simulink model "PTn_model_Z1"  (R2024a)
settings: Solver=ode45  StartTime=0.0  StopTime=20.0  FixedStep=1e-2  RelTol=1e-4  AbsTol=1e-4
values from neighbouring files (symbols this model uses):
  den = [1, 2*D, 1]    [ITAE_Plots_PT2_Schwingfaehig.m]    (also in ITAE_Plots_PTn.m = den_list{i})
  Kp = pid_params{i,j}(1)    [ITAE_Plots_PT2_Schwingfaehig.m]    (also in ITAE_Plots_PTn.m)
  lower_limit = limits(j,2)    [ITAE_Plots_PT2_Schwingfaehig.m]    (also in ITAE_Plots_PTn.m)
  num = [1]    [ITAE_Plots_PT2_Schwingfaehig.m]    (also in ITAE_Plots_PTn.m)
  Tn = pid_params{i,j}(2)    [ITAE_Plots_PT2_Schwingfaehig.m]    (also in ITAE_Plots_PTn.m)
  Tv = pid_params{i,j}(3)    [ITAE_Plots_PT2_Schwingfaehig.m]    (also in ITAE_Plots_PTn.m)
  upper_limit = limits(j,1)    [ITAE_Plots_PT2_Schwingfaehig.m]    (also in ITAE_Plots_PTn.m)
settings Model: Creator=bhir  LastModifiedBy=Flo
settings SolverCC: AlgebraicLoopSolver=TrustRegion
settings DataIOCC: ReturnWorkspaceOutputs=off
settings DebuggingCC: UnconnectedInputMsg=warning  UnconnectedOutputMsg=warning  UnconnectedLineMsg=warning  ArithmeticOperatorsInVariantConditions=warning
settings SFSimCC: SimUseLocalCustomCode=off  CustomCodeUndefinedFunction=UseInterfaceOnly
settings RTWCC: RTWUseLocalCustomCode=off  GPUComputeCapability=3.5  DLArmComputeVersion=19.05
settings CodeAppCC: StateflowObjectComments=on

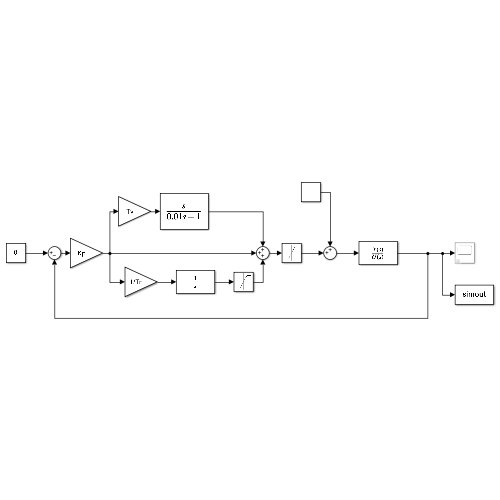
[thumbnail: Simulink's stored preview of the top-level diagram]
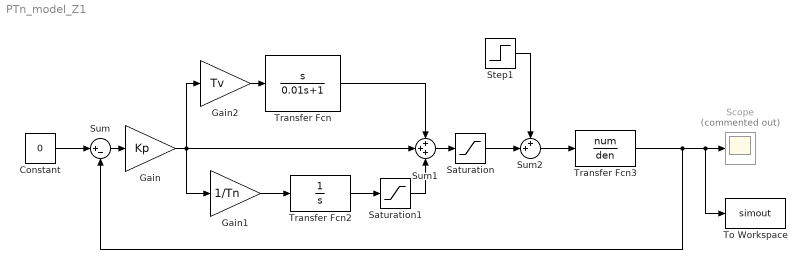
== system PTn_model_Z1 ==
  Constant : Constant  Value=0
  Gain : Gain  Gain=Kp
  Gain1 : Gain  Gain=1/Tn
  Gain2 : Gain  Gain=Tv
  Saturation : Saturate  UpperLimit=upper_limit  LowerLimit=lower_limit
  Saturation1 : Saturate  UpperLimit=upper_limit  LowerLimit=lower_limit
  Scope : Scope  Commented=on
  Step1 : Step  Time=0  SampleTime=0
  Sum : Sum  Inputs=|+-
  Sum1 : Sum  Inputs=+++
  Sum2 : Sum  Inputs=++|
  To Workspace : ToWorkspace  VariableName=simout  SaveFormat=Structure With Time  SampleTime=-1
  Transfer Fcn : TransferFcn  Numerator=[1 0]  Denominator=[0.01 1]
  Transfer Fcn2 : TransferFcn  Denominator=[1 0]
  Transfer Fcn3 : TransferFcn  Numerator=num  Denominator=den
  wires:
  Constant/1 -> Sum/1
  Sum/1 -> Gain/1
  Gain1/1 -> Transfer Fcn2/1
  Sum1/1 -> Saturation/1
  Gain/1 -> Gain2/1, Sum1/2, Gain1/1
  Transfer Fcn/1 -> Sum1/1
  Gain2/1 -> Transfer Fcn/1
  Transfer Fcn3/1 -> Sum/2, To Workspace/1, Scope/1
  Saturation/1 -> Sum2/2
  Transfer Fcn2/1 -> Saturation1/1
  Saturation1/1 -> Sum1/3
  Step1/1 -> Sum2/1
  Sum2/1 -> Transfer Fcn3/1
